simulink model "Pedal_Interpretation_exe"  (Simulink 7.0)
settings: Solver=ode4  StartTime=0.0  StopTime=88  FixedStep=0.01  RelTol=1e-3
InitFcn:
  | PedalInterp_para
values from neighbouring files (symbols this model uses):
  ped_min = 5    [PedalInterp_para.m]
  T_max_Brake = 4000    [PedalInterp_para.m]
  TI = 0    [PAS_callback.m]
undefined symbols (not defined in the file or in its folder): fzgbib, m_ab_100pro, m_ab_70pro, PedalInterpretation, v_bereich
libraries: simulink x320
(part 21 of 23)

== system Pedal_Interpretation_exe/Validation Functions/SR-PI-01.3 Acceleration Pedal recognition/AccPedal == 1/PAS/none - pass - fail/Arbitration/Verdict selection ==
  V1 : Inport  OutDataType=sfix(16)  OutScaling=2^0
  V2 : Inport  Port=2  OutDataType=sfix(16)  OutScaling=2^0
  Delay P F1 F3 : Inport  Port=3  OutDataType=sfix(16)  OutScaling=2^0
  Delay F2 : Inport  Port=4  OutDataType=sfix(16)  OutScaling=2^0
  Delay F4 : Inport  Port=5  OutDataType=sfix(16)  OutScaling=2^0
  Max delay : Inport  Port=6  OutDataType=sfix(16)  OutScaling=2^0
  Compare To Zero1 : simulink/Logic and Bit Operations/Compare To Zero  SystemSampleTime=-1  relop=~=  LogicOutDataTypeMode=boolean  ZeroCross=off
  Constant{2..4,39} (4 alike) : Constant  Value=0  OutDataType=sfix(16)  OutScaling=2^0
  Constant35 : Constant  OutDataType=sfix(16)  OutScaling=2^0
  Constant40 : Constant  Value=2  OutDataType=sfix(16)  OutScaling=2^0
  Memory : Memory
  Memory1 : Memory
  Multiport Switch1 : MultiPortSwitch  Inputs=6  zeroidx=on
  Multiport Switch2 : MultiPortSwitch  Inputs=6  zeroidx=on
  Multiport Switch4 : MultiPortSwitch  Inputs=6  zeroidx=on
  Sum : Sum  OutDataType=sfix(16)  OutScaling=2^0
  Switch : Switch  Criteria=u2 ~= 0
  Switch1 : Switch  Criteria=u2 ~= 0
  Switch2 : Switch  Criteria=u2 ~= 0
  Unit : Constant  OutDataType=sfix(16)  OutScaling=2^0
  Verdict : Outport  OutDataType=sfix(16)  OutScaling=2^0
  Delay : Outport  Port=2  OutDataType=sfix(16)  OutScaling=2^0
  wires:
  Multiport Switch1/1 -> Verdict/1
  Constant39/1 -> Multiport Switch1/7
  Constant2/1 -> Multiport Switch1/6
  Constant3/1 -> Multiport Switch1/5
  Constant4/1 -> Multiport Switch1/4
  Constant35/1 -> Multiport Switch1/3
  Constant40/1 -> Multiport Switch1/2
  V2/1 -> Switch2/3
  V1/1 -> Multiport Switch2/1, Switch/3, Switch2/1
  Max delay/1 -> Multiport Switch2/2, Multiport Switch4/2
  Delay P F1 F3/1 -> Multiport Switch2/3, Multiport Switch2/6, Multiport Switch2/4, Multiport Switch4/6, Multiport Switch4/4, Multiport Switch4/3
  Delay F2/1 -> Multiport Switch2/5, Multiport Switch4/5
  Delay F4/1 -> Multiport Switch2/7, Multiport Switch4/7
  Memory/1 -> Compare To Zero1/1, Switch/1
  Compare To Zero1/1 -> Switch/2, Switch1/2, Switch2/2
  Switch/1 -> Multiport Switch1/1
  Switch1/1 -> Delay/1
  Multiport Switch2/1 -> Switch1/3
  Multiport Switch4/1 -> Memory1/1
  Sum/1 -> Switch1/1
  Memory1/1 -> Sum/2
  Unit/1 -> Sum/1
  Switch2/1 -> Memory/1, Multiport Switch4/1

== system Pedal_Interpretation_exe/Validation Functions/SR-PI-01.3 Acceleration Pedal recognition/AccPedal == 1/PAS/none - pass - fail/Compute delay/Hold1 ==
  " " : Inport  OutDataType=sfix(16)  OutScaling=2^0
  "    " : Inport  Port=2  OutDataType=sfix(16)  OutScaling=2^0
  Memory : Memory  Orientation=left
  Switch : Switch  Criteria=u2 ~= 0
  "  " : Outport  OutDataType=sfix(16)  OutScaling=2^0
  wires:
  Memory/1 -> Switch/3
  Switch/1 -> Memory/1, "  "/1
  "    "/1 -> Switch/1
  " "/1 -> Switch/2

== system Pedal_Interpretation_exe/Validation Functions/SR-PI-01.3 Acceleration Pedal recognition/AccPedal == 1/PAS/none - pass - fail/Compute delay1/Hold1 ==
  " " : Inport  OutDataType=sfix(16)  OutScaling=2^0
  "    " : Inport  Port=2  OutDataType=sfix(16)  OutScaling=2^0
  Memory : Memory  Orientation=left
  Switch : Switch  Criteria=u2 ~= 0
  "  " : Outport  OutDataType=sfix(16)  OutScaling=2^0
  wires:
  Memory/1 -> Switch/3
  Switch/1 -> Memory/1, "  "/1
  "    "/1 -> Switch/1
  " "/1 -> Switch/2

== system Pedal_Interpretation_exe/Validation Functions/SR-PI-01.3 Acceleration Pedal recognition/AccPedal == 1/PAS/none - pass - fail/Compute delay2/Hold1 ==
  " " : Inport  OutDataType=sfix(16)  OutScaling=2^0
  "    " : Inport  Port=2  OutDataType=sfix(16)  OutScaling=2^0
  Memory : Memory  Orientation=left
  Switch : Switch  Criteria=u2 ~= 0
  "  " : Outport  OutDataType=sfix(16)  OutScaling=2^0
  wires:
  " "/1 -> Switch/2
  "    "/1 -> Switch/1
  Switch/1 -> "  "/1, Memory/1
  Memory/1 -> Switch/3

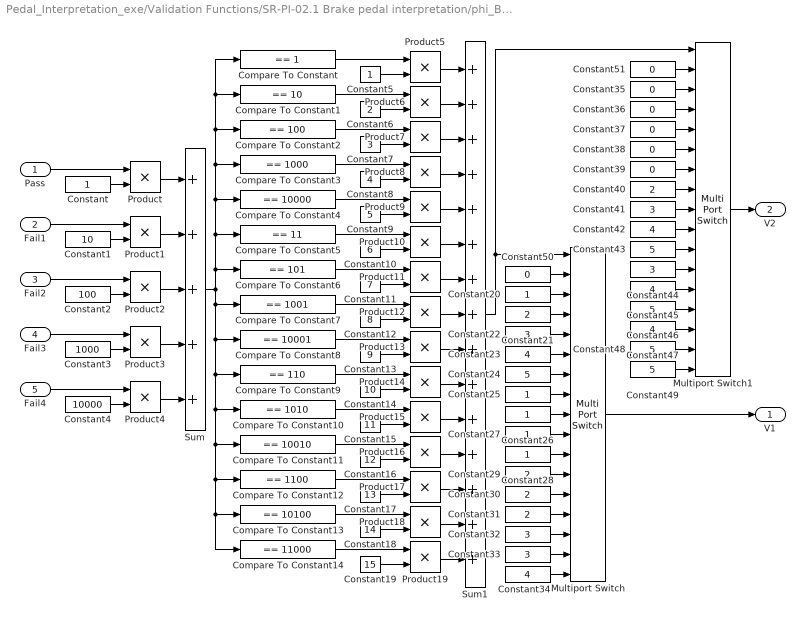
== system Pedal_Interpretation_exe/Validation Functions/SR-PI-02.1 Brake pedal interpretation/phi_Brake/100 = T_des_Brake/T_max_Brake/PAS/none - pass - fail/Arbitration/Verdict identification ==
  Pass : Inport  OutDataType=sfix(16)  OutScaling=2^0
  Fail1 : Inport  Port=2  OutDataType=sfix(16)  OutScaling=2^0
  Fail2 : Inport  Port=3  OutDataType=sfix(16)  OutScaling=2^0
  Fail3 : Inport  Port=4  OutDataType=sfix(16)  OutScaling=2^0
  Fail4 : Inport  Port=5  OutDataType=sfix(16)  OutScaling=2^0
  Compare To Constant : simulink/Logic and Bit Operations/Compare To Constant  SystemSampleTime=-1  relop===  const=1  LogicOutDataTypeMode=uint8  ZeroCross=off
  Compare To Constant1 : simulink/Logic and Bit Operations/Compare To Constant  SystemSampleTime=-1  relop===  const=10  LogicOutDataTypeMode=uint8  ZeroCross=off
  Compare To Constant10 : simulink/Logic and Bit Operations/Compare To Constant  SystemSampleTime=-1  relop===  const=1010  LogicOutDataTypeMode=uint8  ZeroCross=off
  Compare To Constant11 : simulink/Logic and Bit Operations/Compare To Constant  SystemSampleTime=-1  relop===  const=10010  LogicOutDataTypeMode=uint8  ZeroCross=off
  Compare To Constant12 : simulink/Logic and Bit Operations/Compare To Constant  SystemSampleTime=-1  relop===  const=1100  LogicOutDataTypeMode=uint8  ZeroCross=off
  Compare To Constant13 : simulink/Logic and Bit Operations/Compare To Constant  SystemSampleTime=-1  relop===  const=10100  LogicOutDataTypeMode=uint8  ZeroCross=off
  Compare To Constant14 : simulink/Logic and Bit Operations/Compare To Constant  SystemSampleTime=-1  relop===  const=11000  LogicOutDataTypeMode=uint8  ZeroCross=off
  Compare To Constant2 : simulink/Logic and Bit Operations/Compare To Constant  SystemSampleTime=-1  relop===  const=100  LogicOutDataTypeMode=uint8  ZeroCross=off
  Compare To Constant3 : simulink/Logic and Bit Operations/Compare To Constant  SystemSampleTime=-1  relop===  const=1000  LogicOutDataTypeMode=uint8  ZeroCross=off
  Compare To Constant4 : simulink/Logic and Bit Operations/Compare To Constant  SystemSampleTime=-1  relop===  const=10000  LogicOutDataTypeMode=uint8  ZeroCross=off
  Compare To Constant5 : simulink/Logic and Bit Operations/Compare To Constant  SystemSampleTime=-1  relop===  const=11  LogicOutDataTypeMode=uint8  ZeroCross=off
  Compare To Constant6 : simulink/Logic and Bit Operations/Compare To Constant  SystemSampleTime=-1  relop===  const=101  LogicOutDataTypeMode=uint8  ZeroCross=off
  Compare To Constant7 : simulink/Logic and Bit Operations/Compare To Constant  SystemSampleTime=-1  relop===  const=1001  LogicOutDataTypeMode=uint8  ZeroCross=off
  Compare To Constant8 : simulink/Logic and Bit Operations/Compare To Constant  SystemSampleTime=-1  relop===  const=10001  LogicOutDataTypeMode=uint8  ZeroCross=off
  Compare To Constant9 : simulink/Logic and Bit Operations/Compare To Constant  SystemSampleTime=-1  relop===  const=110  LogicOutDataTypeMode=uint8  ZeroCross=off
  Constant{,5,20,25..28} (7 alike) : Constant  OutDataType=sfix(16)  OutScaling=2^0
  Constant1 : Constant  Value=10  OutDataType=sfix(16)  OutScaling=2^0
  Constant10 : Constant  Value=6  OutDataType=sfix(16)  OutScaling=2^0
  Constant11 : Constant  Value=7  OutDataType=sfix(16)  OutScaling=2^0
  Constant12 : Constant  Value=8  OutDataType=sfix(16)  OutScaling=2^0
  Constant13 : Constant  Value=9  OutDataType=sfix(16)  OutScaling=2^0
  Constant14 : Constant  Value=10  OutDataType=sfix(16)  OutScaling=2^0
  Constant15 : Constant  Value=11  OutDataType=sfix(16)  OutScaling=2^0
  Constant16 : Constant  Value=12  OutDataType=sfix(16)  OutScaling=2^0
  Constant17 : Constant  Value=13  OutDataType=sfix(16)  OutScaling=2^0
  Constant18 : Constant  Value=14  OutDataType=sfix(16)  OutScaling=2^0
  Constant19 : Constant  Value=15  OutDataType=sfix(16)  OutScaling=2^0
  Constant2 : Constant  Value=100  OutDataType=sfix(16)  OutScaling=2^0
  Constant{6,21,29..31,40} (6 alike) : Constant  Value=2  OutDataType=sfix(16)  OutScaling=2^0
  Constant{7,22,32..33,41,44} (6 alike) : Constant  Value=3  OutDataType=sfix(16)  OutScaling=2^0
  Constant{8,23,34,42,45,47} (6 alike) : Constant  Value=4  OutDataType=sfix(16)  OutScaling=2^0
  Constant{9,24,43,46,48..49} (6 alike) : Constant  Value=5  OutDataType=sfix(16)  OutScaling=2^0
  Constant3 : Constant  Value=1000  OutDataType=sfix(16)  OutScaling=2^0
  Constant{35..39,50..51} (7 alike) : Constant  Value=0  OutDataType=sfix(16)  OutScaling=2^0
  Constant4 : Constant  Value=10000  OutDataType=sfix(16)  OutScaling=2^0
  Multiport Switch : MultiPortSwitch  Inputs=16  zeroidx=on
  Multiport Switch1 : MultiPortSwitch  Inputs=16  zeroidx=on
  Product{,1..19} (20 alike) : Product  OutDataType=sfix(16)  OutScaling=2^0  RndMeth=Zero
  Sum : Sum  Inputs=+++++  OutDataType=sfix(16)  OutScaling=2^0
  Sum1 : Sum  Inputs=+++++++++++++++  OutDataType=sfix(16)  OutScaling=2^0
  V1 : Outport  OutDataType=sfix(16)  OutScaling=2^0
  V2 : Outport  Port=2  OutDataType=sfix(16)  OutScaling=2^0
  wires:
  Pass/1 -> Product/1
  Fail1/1 -> Product1/1
  Fail2/1 -> Product2/1
  Fail3/1 -> Product3/1
  Fail4/1 -> Product4/1
  Constant3/1 -> Product3/2
  Constant4/1 -> Product4/2
  Constant2/1 -> Product2/2
  Constant1/1 -> Product1/2
  Constant/1 -> Product/2
  Product/1 -> Sum/1
  Product1/1 -> Sum/2
  Product2/1 -> Sum/3
  Product3/1 -> Sum/4
  Product4/1 -> Sum/5
  Compare To Constant/1 -> Product5/1
  Constant5/1 -> Product5/2
  Constant6/1 -> Product6/2
  Compare To Constant1/1 -> Product6/1
  Constant7/1 -> Product7/2
  Constant8/1 -> Product8/2
  Compare To Constant2/1 -> Product7/1
  Compare To Constant3/1 -> Product8/1
  Constant9/1 -> Product9/2
  Compare To Constant4/1 -> Product9/1
  Constant10/1 -> Product10/2
  Compare To Constant5/1 -> Product10/1
  Constant11/1 -> Product11/2
  Compare To Constant6/1 -> Product11/1
  Constant12/1 -> Product12/2
  Compare To Constant7/1 -> Product12/1
  Constant13/1 -> Product13/2
  Compare To Constant8/1 -> Product13/1
  Constant14/1 -> Product14/2
  Compare To Constant9/1 -> Product14/1
  Constant15/1 -> Product15/2
  Compare To Constant10/1 -> Product15/1
  Constant16/1 -> Product16/2
  Compare To Constant11/1 -> Product16/1
  Constant17/1 -> Product17/2
  Compare To Constant12/1 -> Product17/1
  Constant18/1 -> Product18/2
  Compare To Constant13/1 -> Product18/1
  Constant19/1 -> Product19/2
  Compare To Constant14/1 -> Product19/1
  Sum/1 -> Compare To Constant6/1, Compare To Constant5/1, Compare To Constant4/1, Compare To Constant3/1, Compare To Constant2/1, Compare To Constant1/1, Compare To Constant/1, Compare To Constant8/1, Compare To Constant9/1, Compare To Constant10/1, Compare To Constant11/1, Compare To Constant12/1, Compare To Constant14/1, Compare To Constant13/1, Compare To Constant7/1
  Multiport Switch/1 -> V1/1
  Sum1/1 -> Multiport Switch/1, Multiport Switch1/1
  Constant35/1 -> Multiport Switch1/3
  Constant36/1 -> Multiport Switch1/4
  Constant37/1 -> Multiport Switch1/5
  Constant38/1 -> Multiport Switch1/6
  Constant39/1 -> Multiport Switch1/7
  Constant40/1 -> Multiport Switch1/8
  Constant41/1 -> Multiport Switch1/9
  Constant42/1 -> Multiport Switch1/10
  Constant43/1 -> Multiport Switch1/11
  Constant44/1 -> Multiport Switch1/12
  Constant45/1 -> Multiport Switch1/13
  Constant46/1 -> Multiport Switch1/14
  Constant47/1 -> Multiport Switch1/15
  Constant48/1 -> Multiport Switch1/16
  Constant49/1 -> Multiport Switch1/17
  Multiport Switch1/1 -> V2/1
  Product5/1 -> Sum1/1
  Product6/1 -> Sum1/2
  Product7/1 -> Sum1/3
  Product8/1 -> Sum1/4
  Product9/1 -> Sum1/5
  Product10/1 -> Sum1/6
  Product11/1 -> Sum1/7
  Product12/1 -> Sum1/8
  Product13/1 -> Sum1/9
  Product14/1 -> Sum1/10
  Product15/1 -> Sum1/11
  Product16/1 -> Sum1/12
  Product17/1 -> Sum1/13
  Product18/1 -> Sum1/14
  Product19/1 -> Sum1/15
  Constant50/1 -> Multiport Switch/2
  Constant20/1 -> Multiport Switch/3
  Constant21/1 -> Multiport Switch/4
  Constant22/1 -> Multiport Switch/5
  Constant23/1 -> Multiport Switch/6
  Constant24/1 -> Multiport Switch/7
  Constant25/1 -> Multiport Switch/8
  Constant26/1 -> Multiport Switch/9
  Constant27/1 -> Multiport Switch/10
  Constant28/1 -> Multiport Switch/11
  Constant29/1 -> Multiport Switch/12
  Constant30/1 -> Multiport Switch/13
  Constant31/1 -> Multiport Switch/14
  Constant32/1 -> Multiport Switch/15
  Constant33/1 -> Multiport Switch/16
  Constant34/1 -> Multiport Switch/17
  Constant51/1 -> Multiport Switch1/2

== system Pedal_Interpretation_exe/Validation Functions/SR-PI-02.1 Brake pedal interpretation/phi_Brake/100 = T_des_Brake/T_max_Brake/PAS/none - pass - fail/Arbitration/Verdict selection ==
  V1 : Inport  OutDataType=sfix(16)  OutScaling=2^0
  V2 : Inport  Port=2  OutDataType=sfix(16)  OutScaling=2^0
  Delay P F1 F3 : Inport  Port=3  OutDataType=sfix(16)  OutScaling=2^0
  Delay F2 : Inport  Port=4  OutDataType=sfix(16)  OutScaling=2^0
  Delay F4 : Inport  Port=5  OutDataType=sfix(16)  OutScaling=2^0
  Max delay : Inport  Port=6  OutDataType=sfix(16)  OutScaling=2^0
  Compare To Zero1 : simulink/Logic and Bit Operations/Compare To Zero  SystemSampleTime=-1  relop=~=  LogicOutDataTypeMode=boolean  ZeroCross=off
  Constant{2..4,39} (4 alike) : Constant  Value=0  OutDataType=sfix(16)  OutScaling=2^0
  Constant35 : Constant  OutDataType=sfix(16)  OutScaling=2^0
  Constant40 : Constant  Value=2  OutDataType=sfix(16)  OutScaling=2^0
  Memory : Memory
  Memory1 : Memory
  Multiport Switch1 : MultiPortSwitch  Inputs=6  zeroidx=on
  Multiport Switch2 : MultiPortSwitch  Inputs=6  zeroidx=on
  Multiport Switch4 : MultiPortSwitch  Inputs=6  zeroidx=on
  Sum : Sum  OutDataType=sfix(16)  OutScaling=2^0
  Switch : Switch  Criteria=u2 ~= 0
  Switch1 : Switch  Criteria=u2 ~= 0
  Switch2 : Switch  Criteria=u2 ~= 0
  Unit : Constant  OutDataType=sfix(16)  OutScaling=2^0
  Verdict : Outport  OutDataType=sfix(16)  OutScaling=2^0
  Delay : Outport  Port=2  OutDataType=sfix(16)  OutScaling=2^0
  wires:
  Multiport Switch1/1 -> Verdict/1
  Constant39/1 -> Multiport Switch1/7
  Constant2/1 -> Multiport Switch1/6
  Constant3/1 -> Multiport Switch1/5
  Constant4/1 -> Multiport Switch1/4
  Constant35/1 -> Multiport Switch1/3
  Constant40/1 -> Multiport Switch1/2
  V2/1 -> Switch2/3
  V1/1 -> Multiport Switch2/1, Switch/3, Switch2/1
  Max delay/1 -> Multiport Switch2/2, Multiport Switch4/2
  Delay P F1 F3/1 -> Multiport Switch2/3, Multiport Switch2/6, Multiport Switch2/4, Multiport Switch4/6, Multiport Switch4/4, Multiport Switch4/3
  Delay F2/1 -> Multiport Switch2/5, Multiport Switch4/5
  Delay F4/1 -> Multiport Switch2/7, Multiport Switch4/7
  Memory/1 -> Compare To Zero1/1, Switch/1
  Compare To Zero1/1 -> Switch/2, Switch1/2, Switch2/2
  Switch/1 -> Multiport Switch1/1
  Switch1/1 -> Delay/1
  Multiport Switch2/1 -> Switch1/3
  Multiport Switch4/1 -> Memory1/1
  Sum/1 -> Switch1/1
  Memory1/1 -> Sum/2
  Unit/1 -> Sum/1
  Switch2/1 -> Memory/1, Multiport Switch4/1

== system Pedal_Interpretation_exe/Validation Functions/SR-PI-02.1 Brake pedal interpretation/phi_Brake/100 = T_des_Brake/T_max_Brake/PAS/none - pass - fail/Compute delay/Hold1 ==
  " " : Inport  OutDataType=sfix(16)  OutScaling=2^0
  "    " : Inport  Port=2  OutDataType=sfix(16)  OutScaling=2^0
  Memory : Memory  Orientation=left
  Switch : Switch  Criteria=u2 ~= 0
  "  " : Outport  OutDataType=sfix(16)  OutScaling=2^0
  wires:
  Memory/1 -> Switch/3
  Switch/1 -> Memory/1, "  "/1
  "    "/1 -> Switch/1
  " "/1 -> Switch/2

== system Pedal_Interpretation_exe/Validation Functions/SR-PI-02.1 Brake pedal interpretation/phi_Brake/100 = T_des_Brake/T_max_Brake/PAS/none - pass - fail/Compute delay1/Hold1 ==
  " " : Inport  OutDataType=sfix(16)  OutScaling=2^0
  "    " : Inport  Port=2  OutDataType=sfix(16)  OutScaling=2^0
  Memory : Memory  Orientation=left
  Switch : Switch  Criteria=u2 ~= 0
  "  " : Outport  OutDataType=sfix(16)  OutScaling=2^0
  wires:
  Memory/1 -> Switch/3
  Switch/1 -> Memory/1, "  "/1
  "    "/1 -> Switch/1
  " "/1 -> Switch/2

== system Pedal_Interpretation_exe/Validation Functions/SR-PI-02.1 Brake pedal interpretation/phi_Brake/100 = T_des_Brake/T_max_Brake/PAS/none - pass - fail/Compute delay2/Hold1 ==
  " " : Inport  OutDataType=sfix(16)  OutScaling=2^0
  "    " : Inport  Port=2  OutDataType=sfix(16)  OutScaling=2^0
  Memory : Memory  Orientation=left
  Switch : Switch  Criteria=u2 ~= 0
  "  " : Outport  OutDataType=sfix(16)  OutScaling=2^0
  wires:
  " "/1 -> Switch/2
  "    "/1 -> Switch/1
  Switch/1 -> "  "/1, Memory/1
  Memory/1 -> Switch/3

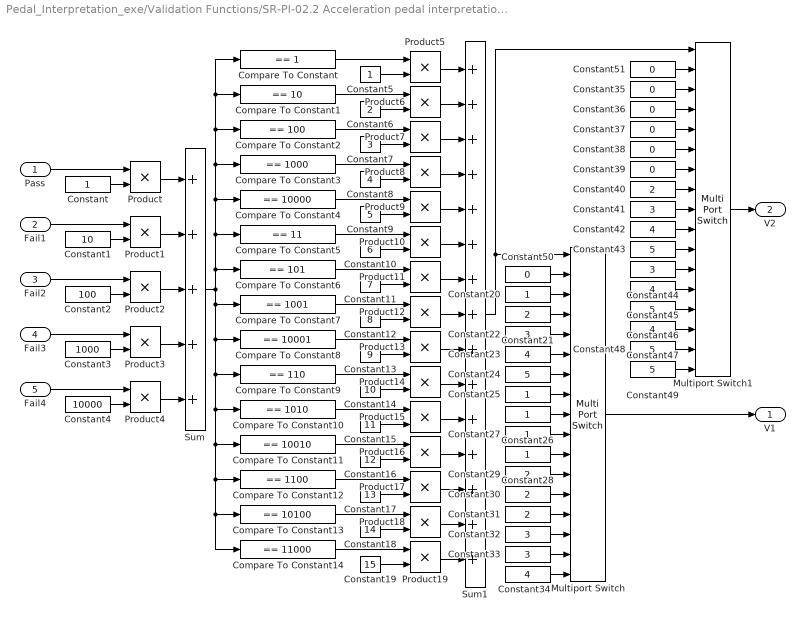
== system Pedal_Interpretation_exe/Validation Functions/SR-PI-02.2 Acceleration pedal interpretation/T_des_Drive = const/PAS/none - pass - fail/Arbitration/Verdict identification ==
  Pass : Inport  OutDataType=sfix(16)  OutScaling=2^0
  Fail1 : Inport  Port=2  OutDataType=sfix(16)  OutScaling=2^0
  Fail2 : Inport  Port=3  OutDataType=sfix(16)  OutScaling=2^0
  Fail3 : Inport  Port=4  OutDataType=sfix(16)  OutScaling=2^0
  Fail4 : Inport  Port=5  OutDataType=sfix(16)  OutScaling=2^0
  Compare To Constant : simulink/Logic and Bit Operations/Compare To Constant  SystemSampleTime=-1  relop===  const=1  LogicOutDataTypeMode=uint8  ZeroCross=off
  Compare To Constant1 : simulink/Logic and Bit Operations/Compare To Constant  SystemSampleTime=-1  relop===  const=10  LogicOutDataTypeMode=uint8  ZeroCross=off
  Compare To Constant10 : simulink/Logic and Bit Operations/Compare To Constant  SystemSampleTime=-1  relop===  const=1010  LogicOutDataTypeMode=uint8  ZeroCross=off
  Compare To Constant11 : simulink/Logic and Bit Operations/Compare To Constant  SystemSampleTime=-1  relop===  const=10010  LogicOutDataTypeMode=uint8  ZeroCross=off
  Compare To Constant12 : simulink/Logic and Bit Operations/Compare To Constant  SystemSampleTime=-1  relop===  const=1100  LogicOutDataTypeMode=uint8  ZeroCross=off
  Compare To Constant13 : simulink/Logic and Bit Operations/Compare To Constant  SystemSampleTime=-1  relop===  const=10100  LogicOutDataTypeMode=uint8  ZeroCross=off
  Compare To Constant14 : simulink/Logic and Bit Operations/Compare To Constant  SystemSampleTime=-1  relop===  const=11000  LogicOutDataTypeMode=uint8  ZeroCross=off
  Compare To Constant2 : simulink/Logic and Bit Operations/Compare To Constant  SystemSampleTime=-1  relop===  const=100  LogicOutDataTypeMode=uint8  ZeroCross=off
  Compare To Constant3 : simulink/Logic and Bit Operations/Compare To Constant  SystemSampleTime=-1  relop===  const=1000  LogicOutDataTypeMode=uint8  ZeroCross=off
  Compare To Constant4 : simulink/Logic and Bit Operations/Compare To Constant  SystemSampleTime=-1  relop===  const=10000  LogicOutDataTypeMode=uint8  ZeroCross=off
  Compare To Constant5 : simulink/Logic and Bit Operations/Compare To Constant  SystemSampleTime=-1  relop===  const=11  LogicOutDataTypeMode=uint8  ZeroCross=off
  Compare To Constant6 : simulink/Logic and Bit Operations/Compare To Constant  SystemSampleTime=-1  relop===  const=101  LogicOutDataTypeMode=uint8  ZeroCross=off
  Compare To Constant7 : simulink/Logic and Bit Operations/Compare To Constant  SystemSampleTime=-1  relop===  const=1001  LogicOutDataTypeMode=uint8  ZeroCross=off
  Compare To Constant8 : simulink/Logic and Bit Operations/Compare To Constant  SystemSampleTime=-1  relop===  const=10001  LogicOutDataTypeMode=uint8  ZeroCross=off
  Compare To Constant9 : simulink/Logic and Bit Operations/Compare To Constant  SystemSampleTime=-1  relop===  const=110  LogicOutDataTypeMode=uint8  ZeroCross=off
  Constant{,5,20,25..28} (7 alike) : Constant  OutDataType=sfix(16)  OutScaling=2^0
  Constant1 : Constant  Value=10  OutDataType=sfix(16)  OutScaling=2^0
  Constant10 : Constant  Value=6  OutDataType=sfix(16)  OutScaling=2^0
  Constant11 : Constant  Value=7  OutDataType=sfix(16)  OutScaling=2^0
  Constant12 : Constant  Value=8  OutDataType=sfix(16)  OutScaling=2^0
  Constant13 : Constant  Value=9  OutDataType=sfix(16)  OutScaling=2^0
  Constant14 : Constant  Value=10  OutDataType=sfix(16)  OutScaling=2^0
  Constant15 : Constant  Value=11  OutDataType=sfix(16)  OutScaling=2^0
  Constant16 : Constant  Value=12  OutDataType=sfix(16)  OutScaling=2^0
  Constant17 : Constant  Value=13  OutDataType=sfix(16)  OutScaling=2^0
  Constant18 : Constant  Value=14  OutDataType=sfix(16)  OutScaling=2^0
  Constant19 : Constant  Value=15  OutDataType=sfix(16)  OutScaling=2^0
  Constant2 : Constant  Value=100  OutDataType=sfix(16)  OutScaling=2^0
  Constant{6,21,29..31,40} (6 alike) : Constant  Value=2  OutDataType=sfix(16)  OutScaling=2^0
  Constant{7,22,32..33,41,44} (6 alike) : Constant  Value=3  OutDataType=sfix(16)  OutScaling=2^0
  Constant{8,23,34,42,45,47} (6 alike) : Constant  Value=4  OutDataType=sfix(16)  OutScaling=2^0
  Constant{9,24,43,46,48..49} (6 alike) : Constant  Value=5  OutDataType=sfix(16)  OutScaling=2^0
  Constant3 : Constant  Value=1000  OutDataType=sfix(16)  OutScaling=2^0
  Constant{35..39,50..51} (7 alike) : Constant  Value=0  OutDataType=sfix(16)  OutScaling=2^0
  Constant4 : Constant  Value=10000  OutDataType=sfix(16)  OutScaling=2^0
  Multiport Switch : MultiPortSwitch  Inputs=16  zeroidx=on
  Multiport Switch1 : MultiPortSwitch  Inputs=16  zeroidx=on
  Product{,1..19} (20 alike) : Product  OutDataType=sfix(16)  OutScaling=2^0  RndMeth=Zero
  Sum : Sum  Inputs=+++++  OutDataType=sfix(16)  OutScaling=2^0
  Sum1 : Sum  Inputs=+++++++++++++++  OutDataType=sfix(16)  OutScaling=2^0
  V1 : Outport  OutDataType=sfix(16)  OutScaling=2^0
  V2 : Outport  Port=2  OutDataType=sfix(16)  OutScaling=2^0
  wires:
  Pass/1 -> Product/1
  Fail1/1 -> Product1/1
  Fail2/1 -> Product2/1
  Fail3/1 -> Product3/1
  Fail4/1 -> Product4/1
  Constant3/1 -> Product3/2
  Constant4/1 -> Product4/2
  Constant2/1 -> Product2/2
  Constant1/1 -> Product1/2
  Constant/1 -> Product/2
  Product/1 -> Sum/1
  Product1/1 -> Sum/2
  Product2/1 -> Sum/3
  Product3/1 -> Sum/4
  Product4/1 -> Sum/5
  Compare To Constant/1 -> Product5/1
  Constant5/1 -> Product5/2
  Constant6/1 -> Product6/2
  Compare To Constant1/1 -> Product6/1
  Constant7/1 -> Product7/2
  Constant8/1 -> Product8/2
  Compare To Constant2/1 -> Product7/1
  Compare To Constant3/1 -> Product8/1
  Constant9/1 -> Product9/2
  Compare To Constant4/1 -> Product9/1
  Constant10/1 -> Product10/2
  Compare To Constant5/1 -> Product10/1
  Constant11/1 -> Product11/2
  Compare To Constant6/1 -> Product11/1
  Constant12/1 -> Product12/2
  Compare To Constant7/1 -> Product12/1
  Constant13/1 -> Product13/2
  Compare To Constant8/1 -> Product13/1
  Constant14/1 -> Product14/2
  Compare To Constant9/1 -> Product14/1
  Constant15/1 -> Product15/2
  Compare To Constant10/1 -> Product15/1
  Constant16/1 -> Product16/2
  Compare To Constant11/1 -> Product16/1
  Constant17/1 -> Product17/2
  Compare To Constant12/1 -> Product17/1
  Constant18/1 -> Product18/2
  Compare To Constant13/1 -> Product18/1
  Constant19/1 -> Product19/2
  Compare To Constant14/1 -> Product19/1
  Sum/1 -> Compare To Constant6/1, Compare To Constant5/1, Compare To Constant4/1, Compare To Constant3/1, Compare To Constant2/1, Compare To Constant1/1, Compare To Constant/1, Compare To Constant8/1, Compare To Constant9/1, Compare To Constant10/1, Compare To Constant11/1, Compare To Constant12/1, Compare To Constant14/1, Compare To Constant13/1, Compare To Constant7/1
  Multiport Switch/1 -> V1/1
  Sum1/1 -> Multiport Switch/1, Multiport Switch1/1
  Constant35/1 -> Multiport Switch1/3
  Constant36/1 -> Multiport Switch1/4
  Constant37/1 -> Multiport Switch1/5
  Constant38/1 -> Multiport Switch1/6
  Constant39/1 -> Multiport Switch1/7
  Constant40/1 -> Multiport Switch1/8
  Constant41/1 -> Multiport Switch1/9
  Constant42/1 -> Multiport Switch1/10
  Constant43/1 -> Multiport Switch1/11
  Constant44/1 -> Multiport Switch1/12
  Constant45/1 -> Multiport Switch1/13
  Constant46/1 -> Multiport Switch1/14
  Constant47/1 -> Multiport Switch1/15
  Constant48/1 -> Multiport Switch1/16
  Constant49/1 -> Multiport Switch1/17
  Multiport Switch1/1 -> V2/1
  Product5/1 -> Sum1/1
  Product6/1 -> Sum1/2
  Product7/1 -> Sum1/3
  Product8/1 -> Sum1/4
  Product9/1 -> Sum1/5
  Product10/1 -> Sum1/6
  Product11/1 -> Sum1/7
  Product12/1 -> Sum1/8
  Product13/1 -> Sum1/9
  Product14/1 -> Sum1/10
  Product15/1 -> Sum1/11
  Product16/1 -> Sum1/12
  Product17/1 -> Sum1/13
  Product18/1 -> Sum1/14
  Product19/1 -> Sum1/15
  Constant50/1 -> Multiport Switch/2
  Constant20/1 -> Multiport Switch/3
  Constant21/1 -> Multiport Switch/4
  Constant22/1 -> Multiport Switch/5
  Constant23/1 -> Multiport Switch/6
  Constant24/1 -> Multiport Switch/7
  Constant25/1 -> Multiport Switch/8
  Constant26/1 -> Multiport Switch/9
  Constant27/1 -> Multiport Switch/10
  Constant28/1 -> Multiport Switch/11
  Constant29/1 -> Multiport Switch/12
  Constant30/1 -> Multiport Switch/13
  Constant31/1 -> Multiport Switch/14
  Constant32/1 -> Multiport Switch/15
  Constant33/1 -> Multiport Switch/16
  Constant34/1 -> Multiport Switch/17
  Constant51/1 -> Multiport Switch1/2

== system Pedal_Interpretation_exe/Validation Functions/SR-PI-02.2 Acceleration pedal interpretation/T_des_Drive = const/PAS/none - pass - fail/Arbitration/Verdict selection ==
  V1 : Inport  OutDataType=sfix(16)  OutScaling=2^0
  V2 : Inport  Port=2  OutDataType=sfix(16)  OutScaling=2^0
  Delay P F1 F3 : Inport  Port=3  OutDataType=sfix(16)  OutScaling=2^0
  Delay F2 : Inport  Port=4  OutDataType=sfix(16)  OutScaling=2^0
  Delay F4 : Inport  Port=5  OutDataType=sfix(16)  OutScaling=2^0
  Max delay : Inport  Port=6  OutDataType=sfix(16)  OutScaling=2^0
  Compare To Zero1 : simulink/Logic and Bit Operations/Compare To Zero  SystemSampleTime=-1  relop=~=  LogicOutDataTypeMode=boolean  ZeroCross=off
  Constant{2..4,39} (4 alike) : Constant  Value=0  OutDataType=sfix(16)  OutScaling=2^0
  Constant35 : Constant  OutDataType=sfix(16)  OutScaling=2^0
  Constant40 : Constant  Value=2  OutDataType=sfix(16)  OutScaling=2^0
  Memory : Memory
  Memory1 : Memory
  Multiport Switch1 : MultiPortSwitch  Inputs=6  zeroidx=on
  Multiport Switch2 : MultiPortSwitch  Inputs=6  zeroidx=on
  Multiport Switch4 : MultiPortSwitch  Inputs=6  zeroidx=on
  Sum : Sum  OutDataType=sfix(16)  OutScaling=2^0
  Switch : Switch  Criteria=u2 ~= 0
  Switch1 : Switch  Criteria=u2 ~= 0
  Switch2 : Switch  Criteria=u2 ~= 0
  Unit : Constant  OutDataType=sfix(16)  OutScaling=2^0
  Verdict : Outport  OutDataType=sfix(16)  OutScaling=2^0
  Delay : Outport  Port=2  OutDataType=sfix(16)  OutScaling=2^0
  wires:
  Multiport Switch1/1 -> Verdict/1
  Constant39/1 -> Multiport Switch1/7
  Constant2/1 -> Multiport Switch1/6
  Constant3/1 -> Multiport Switch1/5
  Constant4/1 -> Multiport Switch1/4
  Constant35/1 -> Multiport Switch1/3
  Constant40/1 -> Multiport Switch1/2
  V2/1 -> Switch2/3
  V1/1 -> Multiport Switch2/1, Switch/3, Switch2/1
  Max delay/1 -> Multiport Switch2/2, Multiport Switch4/2
  Delay P F1 F3/1 -> Multiport Switch2/3, Multiport Switch2/6, Multiport Switch2/4, Multiport Switch4/6, Multiport Switch4/4, Multiport Switch4/3
  Delay F2/1 -> Multiport Switch2/5, Multiport Switch4/5
  Delay F4/1 -> Multiport Switch2/7, Multiport Switch4/7
  Memory/1 -> Compare To Zero1/1, Switch/1
  Compare To Zero1/1 -> Switch/2, Switch1/2, Switch2/2
  Switch/1 -> Multiport Switch1/1
  Switch1/1 -> Delay/1
  Multiport Switch2/1 -> Switch1/3
  Multiport Switch4/1 -> Memory1/1
  Sum/1 -> Switch1/1
  Memory1/1 -> Sum/2
  Unit/1 -> Sum/1
  Switch2/1 -> Memory/1, Multiport Switch4/1

== system Pedal_Interpretation_exe/Validation Functions/SR-PI-02.2 Acceleration pedal interpretation/T_des_Drive = const/PAS/none - pass - fail/Compute delay/Hold1 ==
  " " : Inport  OutDataType=sfix(16)  OutScaling=2^0
  "    " : Inport  Port=2  OutDataType=sfix(16)  OutScaling=2^0
  Memory : Memory  Orientation=left
  Switch : Switch  Criteria=u2 ~= 0
  "  " : Outport  OutDataType=sfix(16)  OutScaling=2^0
  wires:
  Memory/1 -> Switch/3
  Switch/1 -> Memory/1, "  "/1
  "    "/1 -> Switch/1
  " "/1 -> Switch/2

== system Pedal_Interpretation_exe/Validation Functions/SR-PI-02.2 Acceleration pedal interpretation/T_des_Drive = const/PAS/none - pass - fail/Compute delay1/Hold1 ==
  " " : Inport  OutDataType=sfix(16)  OutScaling=2^0
  "    " : Inport  Port=2  OutDataType=sfix(16)  OutScaling=2^0
  Memory : Memory  Orientation=left
  Switch : Switch  Criteria=u2 ~= 0
  "  " : Outport  OutDataType=sfix(16)  OutScaling=2^0
  wires:
  Memory/1 -> Switch/3
  Switch/1 -> Memory/1, "  "/1
  "    "/1 -> Switch/1
  " "/1 -> Switch/2

== system Pedal_Interpretation_exe/Validation Functions/SR-PI-02.2 Acceleration pedal interpretation/T_des_Drive = const/PAS/none - pass - fail/Compute delay2/Hold1 ==
  " " : Inport  OutDataType=sfix(16)  OutScaling=2^0
  "    " : Inport  Port=2  OutDataType=sfix(16)  OutScaling=2^0
  Memory : Memory  Orientation=left
  Switch : Switch  Criteria=u2 ~= 0
  "  " : Outport  OutDataType=sfix(16)  OutScaling=2^0
  wires:
  " "/1 -> Switch/2
  "    "/1 -> Switch/1
  Switch/1 -> "  "/1, Memory/1
  Memory/1 -> Switch/3

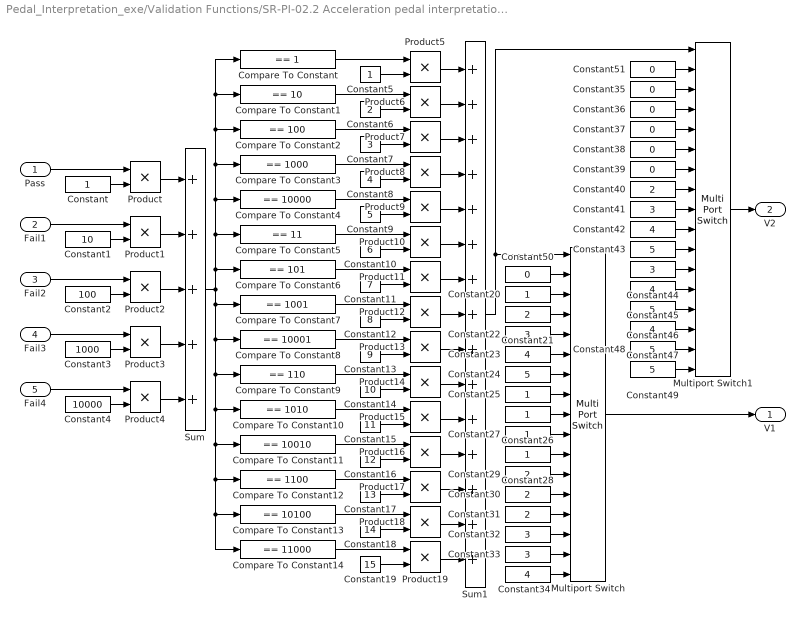
== system Pedal_Interpretation_exe/Validation Functions/SR-PI-02.2 Acceleration pedal interpretation/T_des_Drive decreases/PAS/none - pass - fail/Arbitration/Verdict identification ==
  Pass : Inport  OutDataType=sfix(16)  OutScaling=2^0
  Fail1 : Inport  Port=2  OutDataType=sfix(16)  OutScaling=2^0
  Fail2 : Inport  Port=3  OutDataType=sfix(16)  OutScaling=2^0
  Fail3 : Inport  Port=4  OutDataType=sfix(16)  OutScaling=2^0
  Fail4 : Inport  Port=5  OutDataType=sfix(16)  OutScaling=2^0
  Compare To Constant : simulink/Logic and Bit Operations/Compare To Constant  SystemSampleTime=-1  relop===  const=1  LogicOutDataTypeMode=uint8  ZeroCross=off
  Compare To Constant1 : simulink/Logic and Bit Operations/Compare To Constant  SystemSampleTime=-1  relop===  const=10  LogicOutDataTypeMode=uint8  ZeroCross=off
  Compare To Constant10 : simulink/Logic and Bit Operations/Compare To Constant  SystemSampleTime=-1  relop===  const=1010  LogicOutDataTypeMode=uint8  ZeroCross=off
  Compare To Constant11 : simulink/Logic and Bit Operations/Compare To Constant  SystemSampleTime=-1  relop===  const=10010  LogicOutDataTypeMode=uint8  ZeroCross=off
  Compare To Constant12 : simulink/Logic and Bit Operations/Compare To Constant  SystemSampleTime=-1  relop===  const=1100  LogicOutDataTypeMode=uint8  ZeroCross=off
  Compare To Constant13 : simulink/Logic and Bit Operations/Compare To Constant  SystemSampleTime=-1  relop===  const=10100  LogicOutDataTypeMode=uint8  ZeroCross=off
  Compare To Constant14 : simulink/Logic and Bit Operations/Compare To Constant  SystemSampleTime=-1  relop===  const=11000  LogicOutDataTypeMode=uint8  ZeroCross=off
  Compare To Constant2 : simulink/Logic and Bit Operations/Compare To Constant  SystemSampleTime=-1  relop===  const=100  LogicOutDataTypeMode=uint8  ZeroCross=off
  Compare To Constant3 : simulink/Logic and Bit Operations/Compare To Constant  SystemSampleTime=-1  relop===  const=1000  LogicOutDataTypeMode=uint8  ZeroCross=off
  Compare To Constant4 : simulink/Logic and Bit Operations/Compare To Constant  SystemSampleTime=-1  relop===  const=10000  LogicOutDataTypeMode=uint8  ZeroCross=off
  Compare To Constant5 : simulink/Logic and Bit Operations/Compare To Constant  SystemSampleTime=-1  relop===  const=11  LogicOutDataTypeMode=uint8  ZeroCross=off
  Compare To Constant6 : simulink/Logic and Bit Operations/Compare To Constant  SystemSampleTime=-1  relop===  const=101  LogicOutDataTypeMode=uint8  ZeroCross=off
  Compare To Constant7 : simulink/Logic and Bit Operations/Compare To Constant  SystemSampleTime=-1  relop===  const=1001  LogicOutDataTypeMode=uint8  ZeroCross=off
  Compare To Constant8 : simulink/Logic and Bit Operations/Compare To Constant  SystemSampleTime=-1  relop===  const=10001  LogicOutDataTypeMode=uint8  ZeroCross=off
  Compare To Constant9 : simulink/Logic and Bit Operations/Compare To Constant  SystemSampleTime=-1  relop===  const=110  LogicOutDataTypeMode=uint8  ZeroCross=off
  Constant{,5,20,25..28} (7 alike) : Constant  OutDataType=sfix(16)  OutScaling=2^0
  Constant1 : Constant  Value=10  OutDataType=sfix(16)  OutScaling=2^0
  Constant10 : Constant  Value=6  OutDataType=sfix(16)  OutScaling=2^0
  Constant11 : Constant  Value=7  OutDataType=sfix(16)  OutScaling=2^0
  Constant12 : Constant  Value=8  OutDataType=sfix(16)  OutScaling=2^0
  Constant13 : Constant  Value=9  OutDataType=sfix(16)  OutScaling=2^0
  Constant14 : Constant  Value=10  OutDataType=sfix(16)  OutScaling=2^0
  Constant15 : Constant  Value=11  OutDataType=sfix(16)  OutScaling=2^0
  Constant16 : Constant  Value=12  OutDataType=sfix(16)  OutScaling=2^0
  Constant17 : Constant  Value=13  OutDataType=sfix(16)  OutScaling=2^0
  Constant18 : Constant  Value=14  OutDataType=sfix(16)  OutScaling=2^0
  Constant19 : Constant  Value=15  OutDataType=sfix(16)  OutScaling=2^0
  Constant2 : Constant  Value=100  OutDataType=sfix(16)  OutScaling=2^0
  Constant{6,21,29..31,40} (6 alike) : Constant  Value=2  OutDataType=sfix(16)  OutScaling=2^0
  Constant{7,22,32..33,41,44} (6 alike) : Constant  Value=3  OutDataType=sfix(16)  OutScaling=2^0
  Constant{8,23,34,42,45,47} (6 alike) : Constant  Value=4  OutDataType=sfix(16)  OutScaling=2^0
  Constant{9,24,43,46,48..49} (6 alike) : Constant  Value=5  OutDataType=sfix(16)  OutScaling=2^0
  Constant3 : Constant  Value=1000  OutDataType=sfix(16)  OutScaling=2^0
  Constant{35..39,50..51} (7 alike) : Constant  Value=0  OutDataType=sfix(16)  OutScaling=2^0
  Constant4 : Constant  Value=10000  OutDataType=sfix(16)  OutScaling=2^0
  Multiport Switch : MultiPortSwitch  Inputs=16  zeroidx=on
  Multiport Switch1 : MultiPortSwitch  Inputs=16  zeroidx=on
  Product{,1..19} (20 alike) : Product  OutDataType=sfix(16)  OutScaling=2^0  RndMeth=Zero
  Sum : Sum  Inputs=+++++  OutDataType=sfix(16)  OutScaling=2^0
  Sum1 : Sum  Inputs=+++++++++++++++  OutDataType=sfix(16)  OutScaling=2^0
  V1 : Outport  OutDataType=sfix(16)  OutScaling=2^0
  V2 : Outport  Port=2  OutDataType=sfix(16)  OutScaling=2^0
  wires:
  Pass/1 -> Product/1
  Fail1/1 -> Product1/1
  Fail2/1 -> Product2/1
  Fail3/1 -> Product3/1
  Fail4/1 -> Product4/1
  Constant3/1 -> Product3/2
  Constant4/1 -> Product4/2
  Constant2/1 -> Product2/2
  Constant1/1 -> Product1/2
  Constant/1 -> Product/2
  Product/1 -> Sum/1
  Product1/1 -> Sum/2
  Product2/1 -> Sum/3
  Product3/1 -> Sum/4
  Product4/1 -> Sum/5
  Compare To Constant/1 -> Product5/1
  Constant5/1 -> Product5/2
  Constant6/1 -> Product6/2
  Compare To Constant1/1 -> Product6/1
  Constant7/1 -> Product7/2
  Constant8/1 -> Product8/2
  Compare To Constant2/1 -> Product7/1
  Compare To Constant3/1 -> Product8/1
  Constant9/1 -> Product9/2
  Compare To Constant4/1 -> Product9/1
  Constant10/1 -> Product10/2
  Compare To Constant5/1 -> Product10/1
  Constant11/1 -> Product11/2
  Compare To Constant6/1 -> Product11/1
  Constant12/1 -> Product12/2
  Compare To Constant7/1 -> Product12/1
  Constant13/1 -> Product13/2
  Compare To Constant8/1 -> Product13/1
  Constant14/1 -> Product14/2
  Compare To Constant9/1 -> Product14/1
  Constant15/1 -> Product15/2
  Compare To Constant10/1 -> Product15/1
  Constant16/1 -> Product16/2
  Compare To Constant11/1 -> Product16/1
  Constant17/1 -> Product17/2
  Compare To Constant12/1 -> Product17/1
  Constant18/1 -> Product18/2
  Compare To Constant13/1 -> Product18/1
  Constant19/1 -> Product19/2
  Compare To Constant14/1 -> Product19/1
  Sum/1 -> Compare To Constant6/1, Compare To Constant5/1, Compare To Constant4/1, Compare To Constant3/1, Compare To Constant2/1, Compare To Constant1/1, Compare To Constant/1, Compare To Constant8/1, Compare To Constant9/1, Compare To Constant10/1, Compare To Constant11/1, Compare To Constant12/1, Compare To Constant14/1, Compare To Constant13/1, Compare To Constant7/1
  Multiport Switch/1 -> V1/1
  Sum1/1 -> Multiport Switch/1, Multiport Switch1/1
  Constant35/1 -> Multiport Switch1/3
  Constant36/1 -> Multiport Switch1/4
  Constant37/1 -> Multiport Switch1/5
  Constant38/1 -> Multiport Switch1/6
  Constant39/1 -> Multiport Switch1/7
  Constant40/1 -> Multiport Switch1/8
  Constant41/1 -> Multiport Switch1/9
  Constant42/1 -> Multiport Switch1/10
  Constant43/1 -> Multiport Switch1/11
  Constant44/1 -> Multiport Switch1/12
  Constant45/1 -> Multiport Switch1/13
  Constant46/1 -> Multiport Switch1/14
  Constant47/1 -> Multiport Switch1/15
  Constant48/1 -> Multiport Switch1/16
  Constant49/1 -> Multiport Switch1/17
  Multiport Switch1/1 -> V2/1
  Product5/1 -> Sum1/1
  Product6/1 -> Sum1/2
  Product7/1 -> Sum1/3
  Product8/1 -> Sum1/4
  Product9/1 -> Sum1/5
  Product10/1 -> Sum1/6
  Product11/1 -> Sum1/7
  Product12/1 -> Sum1/8
  Product13/1 -> Sum1/9
  Product14/1 -> Sum1/10
  Product15/1 -> Sum1/11
  Product16/1 -> Sum1/12
  Product17/1 -> Sum1/13
  Product18/1 -> Sum1/14
  Product19/1 -> Sum1/15
  Constant50/1 -> Multiport Switch/2
  Constant20/1 -> Multiport Switch/3
  Constant21/1 -> Multiport Switch/4
  Constant22/1 -> Multiport Switch/5
  Constant23/1 -> Multiport Switch/6
  Constant24/1 -> Multiport Switch/7
  Constant25/1 -> Multiport Switch/8
  Constant26/1 -> Multiport Switch/9
  Constant27/1 -> Multiport Switch/10
  Constant28/1 -> Multiport Switch/11
  Constant29/1 -> Multiport Switch/12
  Constant30/1 -> Multiport Switch/13
  Constant31/1 -> Multiport Switch/14
  Constant32/1 -> Multiport Switch/15
  Constant33/1 -> Multiport Switch/16
  Constant34/1 -> Multiport Switch/17
  Constant51/1 -> Multiport Switch1/2

== system Pedal_Interpretation_exe/Validation Functions/SR-PI-02.2 Acceleration pedal interpretation/T_des_Drive decreases/PAS/none - pass - fail/Arbitration/Verdict selection ==
  V1 : Inport  OutDataType=sfix(16)  OutScaling=2^0
  V2 : Inport  Port=2  OutDataType=sfix(16)  OutScaling=2^0
  Delay P F1 F3 : Inport  Port=3  OutDataType=sfix(16)  OutScaling=2^0
  Delay F2 : Inport  Port=4  OutDataType=sfix(16)  OutScaling=2^0
  Delay F4 : Inport  Port=5  OutDataType=sfix(16)  OutScaling=2^0
  Max delay : Inport  Port=6  OutDataType=sfix(16)  OutScaling=2^0
  Compare To Zero1 : simulink/Logic and Bit Operations/Compare To Zero  SystemSampleTime=-1  relop=~=  LogicOutDataTypeMode=boolean  ZeroCross=off
  Constant{2..4,39} (4 alike) : Constant  Value=0  OutDataType=sfix(16)  OutScaling=2^0
  Constant35 : Constant  OutDataType=sfix(16)  OutScaling=2^0
  Constant40 : Constant  Value=2  OutDataType=sfix(16)  OutScaling=2^0
  Memory : Memory
  Memory1 : Memory
  Multiport Switch1 : MultiPortSwitch  Inputs=6  zeroidx=on
  Multiport Switch2 : MultiPortSwitch  Inputs=6  zeroidx=on
  Multiport Switch4 : MultiPortSwitch  Inputs=6  zeroidx=on
  Sum : Sum  OutDataType=sfix(16)  OutScaling=2^0
  Switch : Switch  Criteria=u2 ~= 0
  Switch1 : Switch  Criteria=u2 ~= 0
  Switch2 : Switch  Criteria=u2 ~= 0
  Unit : Constant  OutDataType=sfix(16)  OutScaling=2^0
  Verdict : Outport  OutDataType=sfix(16)  OutScaling=2^0
  Delay : Outport  Port=2  OutDataType=sfix(16)  OutScaling=2^0
  wires:
  Multiport Switch1/1 -> Verdict/1
  Constant39/1 -> Multiport Switch1/7
  Constant2/1 -> Multiport Switch1/6
  Constant3/1 -> Multiport Switch1/5
  Constant4/1 -> Multiport Switch1/4
  Constant35/1 -> Multiport Switch1/3
  Constant40/1 -> Multiport Switch1/2
  V2/1 -> Switch2/3
  V1/1 -> Multiport Switch2/1, Switch/3, Switch2/1
  Max delay/1 -> Multiport Switch2/2, Multiport Switch4/2
  Delay P F1 F3/1 -> Multiport Switch2/3, Multiport Switch2/6, Multiport Switch2/4, Multiport Switch4/6, Multiport Switch4/4, Multiport Switch4/3
  Delay F2/1 -> Multiport Switch2/5, Multiport Switch4/5
  Delay F4/1 -> Multiport Switch2/7, Multiport Switch4/7
  Memory/1 -> Compare To Zero1/1, Switch/1
  Compare To Zero1/1 -> Switch/2, Switch1/2, Switch2/2
  Switch/1 -> Multiport Switch1/1
  Switch1/1 -> Delay/1
  Multiport Switch2/1 -> Switch1/3
  Multiport Switch4/1 -> Memory1/1
  Sum/1 -> Switch1/1
  Memory1/1 -> Sum/2
  Unit/1 -> Sum/1
  Switch2/1 -> Memory/1, Multiport Switch4/1

== system Pedal_Interpretation_exe/Validation Functions/SR-PI-02.2 Acceleration pedal interpretation/T_des_Drive decreases/PAS/none - pass - fail/Compute delay/Hold1 ==
  " " : Inport  OutDataType=sfix(16)  OutScaling=2^0
  "    " : Inport  Port=2  OutDataType=sfix(16)  OutScaling=2^0
  Memory : Memory  Orientation=left
  Switch : Switch  Criteria=u2 ~= 0
  "  " : Outport  OutDataType=sfix(16)  OutScaling=2^0
  wires:
  Memory/1 -> Switch/3
  Switch/1 -> Memory/1, "  "/1
  "    "/1 -> Switch/1
  " "/1 -> Switch/2

== system Pedal_Interpretation_exe/Validation Functions/SR-PI-02.2 Acceleration pedal interpretation/T_des_Drive decreases/PAS/none - pass - fail/Compute delay1/Hold1 ==
  " " : Inport  OutDataType=sfix(16)  OutScaling=2^0
  "    " : Inport  Port=2  OutDataType=sfix(16)  OutScaling=2^0
  Memory : Memory  Orientation=left
  Switch : Switch  Criteria=u2 ~= 0
  "  " : Outport  OutDataType=sfix(16)  OutScaling=2^0
  wires:
  Memory/1 -> Switch/3
  Switch/1 -> Memory/1, "  "/1
  "    "/1 -> Switch/1
  " "/1 -> Switch/2

== system Pedal_Interpretation_exe/Validation Functions/SR-PI-02.2 Acceleration pedal interpretation/T_des_Drive decreases/PAS/none - pass - fail/Compute delay2/Hold1 ==
  " " : Inport  OutDataType=sfix(16)  OutScaling=2^0
  "    " : Inport  Port=2  OutDataType=sfix(16)  OutScaling=2^0
  Memory : Memory  Orientation=left
  Switch : Switch  Criteria=u2 ~= 0
  "  " : Outport  OutDataType=sfix(16)  OutScaling=2^0
  wires:
  " "/1 -> Switch/2
  "    "/1 -> Switch/1
  Switch/1 -> "  "/1, Memory/1
  Memory/1 -> Switch/3
